simulink model "AAI"  (R2022a)
settings: Solver=FixedStepAuto  StartTime=0.0  StopTime=50  FixedStep=1e-3  RelTol=1e-3  EnableMultiTasking=on
undefined symbols (not defined in the file): D0, D10, D11, D12, D13, D2, D5, D6, D8, D9, PTA0, PTA2, PTB9, PTC16, PTC2, PTC4, PTD0, PTD1, PTD2, PTD3
libraries: frdmk64flib x10
settings Model: ExtModeTrigDuration=5  Creator=MichaelGolendukhin  LastModifiedBy=MichaelGolendukhin
settings OptimizationCC: EnhancedBackFolding=on  PassReuseOutputArgsAs=Individual arguments  ZeroExternalMemoryAtStartup=off  ZeroInternalMemoryAtStartup=off  MaxStackSize=64  OptimizeBlockOrder=speed  DifferentSizesBufferReuse=on  OptimizationCustomize=off  EfficientTunableParamExpr=on
settings DebuggingCC: ParameterTunabilityLossMsg=error
settings HardwareCC: ProdBitPerPointer=32  ProdBitPerSizeT=32  ProdBitPerPtrDiffT=32  ProdLargestAtomicInteger=Long  ProdLargestAtomicFloat=Double  ProdWordSize=32  ProdHWDeviceType=ARM Compatible->ARM Cortex  UseEmbeddedCoderFeatures=off
settings SFSimCC: MATLABDynamicMemAlloc=off
settings RTWCC: SystemTargetFile=ert.tlc  HardwareBoard=NXP FRDM-K64F  TLCOptions="-aInlineSetEventsForThisBaseRateFcn=TLC_FALSE -aSuppressMultiTaskScheduler=TLC_FALSE  -aRateBasedStepFcn=0"  TemplateMakefile=ert_default_tmf  Toolchain=GNU Tools for ARM Embedded Processors
settings CodeAppCC: ForceParamTrailComments=on  IgnoreCustomStorageClasses=off  OperatorAnnotations=on  SimulinkDataObjDesc=on  SFDataObjDesc=on  InsertBlockDesc=on
settings ERTTargetCC: SupportNonInlinedSFcns=on  ExtModeTransport=4  ExtModeMexFile=sendToCommService

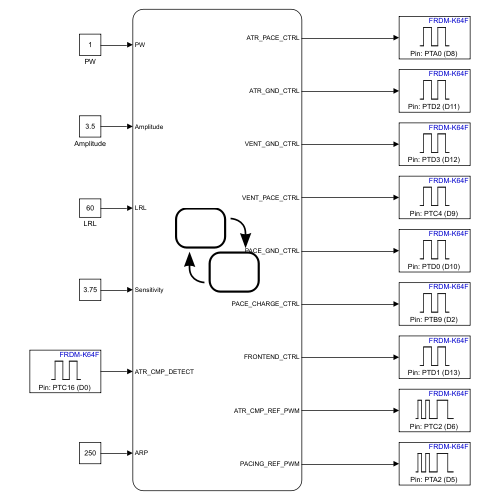
[thumbnail: Simulink's stored preview of the top-level diagram]
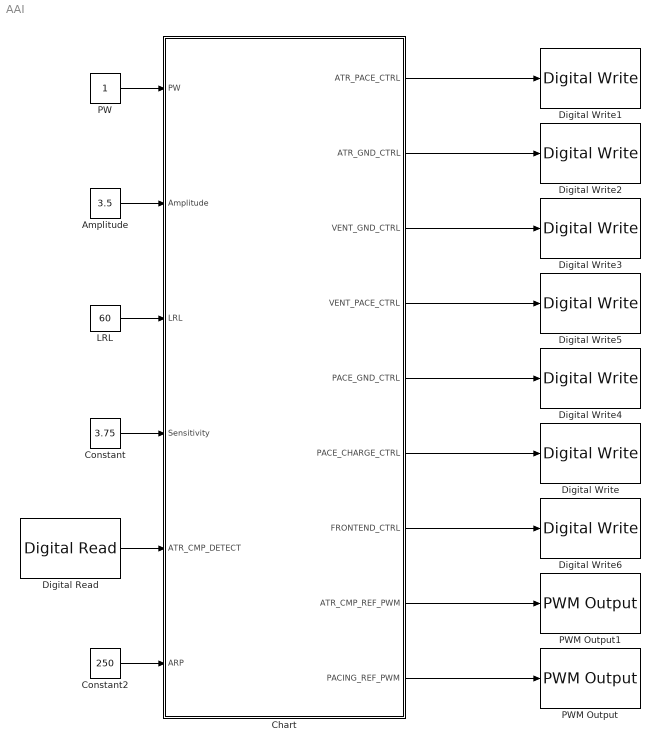
== system AAI ==
  Amplitude : Constant  Value=3.5
  Chart : Stateflow chart  TreatAsAtomicUnit=on
      settings: PortSchema="{\"entries\":[{\"content\":{\"sides\":[{\"content\":{\"connectorIds\":[\"In1\",\"In2\",\"In3\",\"In4\",\"In5\",\"In6\"]},\"type\":\"ConnectorPlacement.EquallySpacedRectSide\",\"uuid\":\"2dca410f-8f43-416b-b245-db6a1c9e2101\"},{\"content\":{\"connectorIds\":[\"Out2\",\"Out1\",\"Out4\",\"Out5\",\"Out6\",\"Out3\",\"Out8\",\"Out9\",\"Out7\"],\"side\":\"RIGHT\"},\"type\":\"ConnectorPlacement.EquallySpacedRectSide\",\"uuid\":\"30508f3d-7d2b-4c80-aa19-382c3c260e83\"},{\"content\":{\"connectorIds\":[],\"side\":\"TOP\"},\"type\":\"ConnectorPlacement.EquallySpacedRectSide\",\"uuid\":\"0cf054d9-a9d5-4fcc-8b60-c098224d8790\"}]},\"type\":\"ConnectorPlacement.EquallySpacedConnector\",\"uuid\":\"125de75b-c166-48e2-8d91-77ead1c82200\"}],\"packageUris\":[\"http://schema.mathworks.com/mf0/Connector/R2020b\"],\"version\":\"1.0\"}"
  Constant : Constant  Value=3.75
  Constant2 : Constant  Value=250
  Digital Read : frdmk64flib/Digital Read  Whichpin=PTC16 (D0)  SampleTime=-1
  Digital Write : frdmk64flib/Digital Write  Whichpin=PTB9 (D2)
  Digital Write1 : frdmk64flib/Digital Write  Whichpin=PTA0 (D8)
  Digital Write2 : frdmk64flib/Digital Write  Whichpin=PTD2 (D11)
  Digital Write3 : frdmk64flib/Digital Write  Whichpin=PTD3 (D12)
  Digital Write4 : frdmk64flib/Digital Write  Whichpin=PTD0 (D10)
  Digital Write5 : frdmk64flib/Digital Write  Whichpin=PTC4 (D9)
  Digital Write6 : frdmk64flib/Digital Write  Whichpin=PTD1 (D13)
  LRL : Constant  Value=60
  PW : Constant
  PWM Output : frdmk64flib/PWM Output  Whichpin=PTA2 (D5)  InitialFrequency=2000  InitialDutyCycle=0
  PWM Output1 : frdmk64flib/PWM Output  Whichpin=PTC2 (D6)  InitialFrequency=2000  InitialDutyCycle=0
  wires:
  PW/1 -> Chart/1(PW)
  LRL/1 -> Chart/3(LRL)
  Chart/2(ATR_PACE_CTRL) -> Digital Write1/1
  Chart/3(PACE_CHARGE_CTRL) -> Digital Write/1
  Chart/1(ATR_GND_CTRL) -> Digital Write2/1
  Chart/4(VENT_GND_CTRL) -> Digital Write3/1
  Chart/5(VENT_PACE_CTRL) -> Digital Write5/1
  Chart/6(PACE_GND_CTRL) -> Digital Write4/1
  Amplitude/1 -> Chart/2(Amplitude)
  Chart/7(PACING_REF_PWM) -> PWM Output/1
  Chart/8(FRONTEND_CTRL) -> Digital Write6/1
  Chart/9(ATR_CMP_REF_PWM) -> PWM Output1/1
  Constant/1 -> Chart/4(Sensitivity)
  Digital Read/1 -> Chart/5(ATR_CMP_DETECT)
  Constant2/1 -> Chart/6(ARP)

== stateflow chart AAI/Chart ==
  state AAI_Charging_C22
    entry:
    VENT_PACE_CTRL = false;
    ATR_PACE_CTRL = false;
    PACE_CHARGE_CTRL = true;
    PACING_REF_PWM = Amplitude * 20;
    PACE_GND_CTRL= true;
    VENT_GND_CTRL = false;
    ATR_GND_CTRL = true;
  state AAI_Pacing
    entry:
    PACE_CHARGE_CTRL = false;
    PACE_GND_CTRL = true;
    VENT_PACE_CTRL = false;
    VENT_GND_CTRL = false;
    ATR_GND_CTRL = false;
    ATR_PACE_CTRL = true;
  state AAI_Sensing
    entry:
    FRONTEND_CTRL = true;
    ATR_CMP_REF_PWM = (Sensitivity)*20;
    exit:
    FRONTEND_CTRL = false;
  (default) -> AAI_Charging_C22
  AAI_Pacing -> AAI_Charging_C22 : after(PW, msec)
  AAI_Sensing -> AAI_Pacing [order 2] : after(((60000/LRL) - ARP), msec)
  AAI_Sensing -> AAI_Charging_C22 [order 1] : [ATR_CMP_DETECT == true]
  AAI_Charging_C22 -> AAI_Sensing : after(ARP, msec)
  data: ATR_GND_CTRL output boolean; ATR_PACE_CTRL output boolean; PACE_CHARGE_CTRL output boolean; VENT_GND_CTRL output boolean; VENT_PACE_CTRL output boolean; PACE_GND_CTRL output boolean; PW input double; Amplitude input double; LRL input double; PACING_REF_PWM output double; Sensitivity input double; FRONTEND_CTRL output boolean; ATR_CMP_DETECT input boolean; ARP input double; ATR_CMP_REF_PWM output double
